simulink model "synchronizing_breaker"  (R2014a)
settings: Solver=FixedStepDiscrete  StartTime=0.0  StopTime=3  FixedStep=Ts  MaxStep=1/60  RelTol=1e-4
PreLoadFcn:
  | load('synchbreaker_data');
StartFcn:
  | tic;
StopFcn:
  | toc;
values from neighbouring files (symbols this model uses):
  d1 = 0.04    [synchbreaker_data.mat]
  Ts = 4e-05    [synchbreaker_data.mat]
libraries: powerlib x11, powerlib_meascontrol x3, simulink x2
settings Model: Creator=gdudgeon  LastModifiedBy=cosorio
settings DataIOCC: SaveOutput=off  SaveTime=off
settings OptimizationCC: ExpressionDepthLimit=2147483647
settings DebuggingCC: UnderspecifiedInitializationDetection=Classic  FcnCallInpInsideContextMsg=UseLocalSettings  StateNameClashWarn=warning
settings SFSimCC: SimParseCustomCode=off
settings GRTTargetCC: CombineOutputUpdateFcns=off  GRTInterface=on

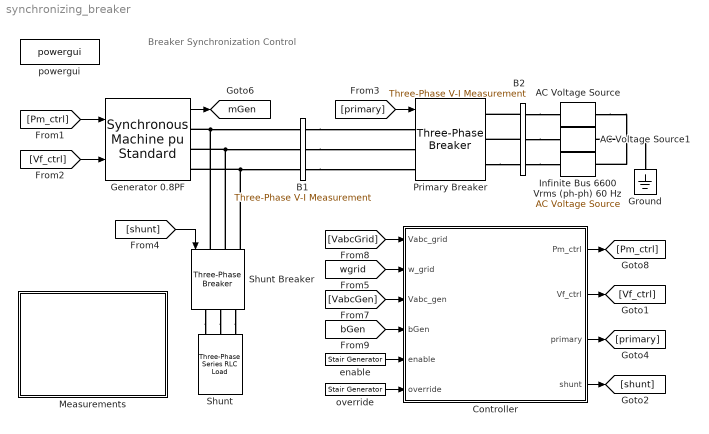
== system synchronizing_breaker ==
  note: Breaker Synchronization Control
  AC Voltage Source : powerlib/Electrical Sources/AC Voltage Source  Amplitude=6600*sqrt(2)/sqrt(3)  Phase=0  Frequency=60  SampleTime=Ts  Measurements=None
  AC Voltage Source1 : powerlib/Electrical Sources/AC Voltage Source  Amplitude=6600*sqrt(2)/sqrt(3)  Phase=-120  Frequency=60  SampleTime=Ts  Measurements=None
  B1 : powerlib/Measurements/Three-Phase V-I Measurement  VoltageMeasurement=phase-to-phase  SetLabelV=on  LabelV=VabcGen  Vpu=off  VpuLL=on  CurrentMeasurement=yes  SetLabelI=on  LabelI=IabcGen  Ipu=on  Pbase=5e6  Vbase=6600  OutputType=Complex  PhasorSimulation=off  PSBequivalent=0
  B2 : powerlib/Measurements/Three-Phase V-I Measurement  VoltageMeasurement=phase-to-phase  SetLabelV=on  LabelV=VabcGrid  Vpu=off  VpuLL=on  CurrentMeasurement=no  SetLabelI=off  LabelI=IabcB2  Ipu=off  Pbase=100e6  Vbase=6600  OutputType=Complex  PhasorSimulation=off  PSBequivalent=0
  Controller : Subsystem  RequirementInfo={'other' 'D:\CVS_Sandbox\P-MLSPG-20171\JIN002 - LPD Modelling\LPD Models\T1702v4_REQM_LINK.doc' '@Simulink_requirement_item_1' 'true' 'Update WR21 automatic synchronisation breaker for use on the LPD model.' '' } %GIDa_fd92f33b_c6ac_4758_9415_28d98727e0ba  TreatAsAtomicUnit=on  SystemSampleTime=Ts
  Generator 0.8PF : powerlib/Machines/Synchronous Machine pu Standard  PresetModel=No  MechanicalLoad=Mechanical power Pm  ShowDetailedParameters=on  RotorType=Salient-pole  Units=per unit standard parameters  MeasurementBus=off  NominalParameters=[5e6 6600 60]  Reactances1=[ 1.81, 0.3, 0.23, 1.76, 0.65, 0.25, 0.15 ]  Reactances2=[1.3050 0.2960 0.2520 0.4740 0.2430 0.1800]  dAxisTimeConstants=Open-circuit  qAxisTimeConstants=Short-circuit  TimeConstants1="[ 4.4849  0.0681  0.1  ]"  TimeConstants2=[ 8.0, 0.03, 1.0, 0.07 ]  TimeConstants3=[4.4900 0.0681 0.0513]  TimeConstants4=[ 8.0, 0.03, 0.3371, 0.0295 ]  TimeConstants5=[ 1.01, 0.053, 0.1 ]  TimeConstants6=[ 1.3201, 0.023, 1.0, 0.07 ]  TimeConstants7=[0.012 0.003 0.003]  TimeConstants8=[ 1.3201, 0.0231, 0.3371, 0.0295 ]  StatorResistance=0.003  Mechanical="[3.7 0.1  4]"  PolePairs=4  InitialConditions=[0 -79.2767 0.4 0.4 0.4 0 -120 120 1.08084]  SetSaturation=off  Saturation=[0.6404,0.7127,0.8441,0.9214,0.9956,1.082,1.19,1.316,1.457;0.7,0.7698,0.8872,0.9466,0.9969,1.046,1.1,1.151,1.201]  LoadFlowParameters=[2 2000000 0 0 0]  TsPowergui=0  TsBlock=-1  IterativeModel=Forward Euler  BusType=swing  Pref=0  Qref=0  Qmin=-inf  Qmax=inf  PLF=0  QLF=0
      settings: AttributesFormatString=%<NominalParameters>
  Ground : powerlib/Elements/Ground  LConnTagsString=a
  Infinite Bus 6600 Vrms (ph-ph) 60 Hz : powerlib/Electrical Sources/AC Voltage Source  Amplitude=6600*sqrt(2)/sqrt(3)  Phase=120  Frequency=60  SampleTime=Ts  Measurements=None
  Measurements : Subsystem
  Primary Breaker : powerlib/Elements/Three-Phase Breaker  InitialState=closed  SwitchA=on  SwitchB=on  SwitchC=on  SwitchTimes="[4/60  10/60]"  External=on  BreakerResistance=1e-5  SnubberResistance=1e6  SnubberCapacitance=Inf  Measurements=None
  Shunt : powerlib/Elements/Three-Phase Series RLC Load  LConnTagsString=A|B|C  Configuration=Y (grounded)  NominalVoltage=6600  NominalFrequency=60  ActivePower=2e5  InductivePower=0  CapacitivePower=0  Measurements=None  LoadType=constant Z
      settings: AttributesFormatString=|
      | P = %<ActivePower> W
      | V = %<NominalVoltage> Vrms
  Shunt Breaker : powerlib/Elements/Three-Phase Breaker  InitialState=open  SwitchA=on  SwitchB=on  SwitchC=on  SwitchTimes="[4/60  10/60]"  External=on  BreakerResistance=1e-5  SnubberResistance=1e6  SnubberCapacitance=Inf  Measurements=None
  enable : powerlib_meascontrol/Pulse & Signal Generators/Stair Generator  t=[0, 1]  e=[0, 1]  Ts=Ts
  override : powerlib_meascontrol/Pulse & Signal Generators/Stair Generator  t=[0, 0.5]  e=[1, 0]  Ts=Ts
  powergui : powerlib/powergui  SimulationMode=Discrete  SolverType=Backward Euler  SampleTime=Ts  frequency=60  SPID=off  DisableSnubberDevices=off  DisableRonSwitches=off  DisableVfSwitches=off  SwTol=0  Interpol=off  DisplayEquations=off  Ts=0  methode=off  frequencyindice=60  Pbase=100e6  ErrMax=1e-4  Iterations=50  UnitsV=kV  UnitsW=MW  FunctionMessages=off  echomessages=off  HookPort=off  EnableUseOfTLC=off  x0status=blocks  RestoreLinks=warning  ResistiveCurrentMeasurement=off  Frange=[0:2:500]  Ylog=off  Xlog=on  ShowGrid=off  save=off  variable=ZData  structure=0  ZoomFFT=on  StartTime=0.0  cycles=1  DisplayStyle=1  fundamental=60  FreqAxis=off  MaxFrequency=1000  frequencyindicesteady=1  RmsSteady=1  display=off
  tag scope: mGen=global
  wires:
  override/1 -> Controller/6(override)
  enable/1 -> Controller/5(enable)
  [Vf_ctrl] -> Generator 0.8PF/2
  [Pm_ctrl] -> Generator 0.8PF/1
  Controller/3(primary) -> [primary]
  [primary] -> Primary Breaker/1
  [shunt] -> Shunt Breaker/1
  Generator 0.8PF/1 -> [mGen]
  [VabcGen] -> Controller/3(Vabc_gen)
  [VabcGrid] -> Controller/1(Vabc_grid)
  [bGen] -> Controller/4(bGen)
  Controller/1(Pm_ctrl) -> [Pm_ctrl]
  Controller/2(Vf_ctrl) -> [Vf_ctrl]
  Controller/4(shunt) -> [shunt]
  [wgrid] -> Controller/2(w_grid)
  connections:
  Shunt Breaker/LConn3 -- B1/LConn3 -- Generator 0.8PF/RConn3
  B2/LConn2 -- Primary Breaker/RConn2
  B1/RConn1 -- Primary Breaker/LConn1
  Shunt Breaker/RConn1 -- Shunt/LConn1
  Shunt Breaker/RConn2 -- Shunt/LConn2
  Shunt Breaker/RConn3 -- Shunt/LConn3
  B2/LConn1 -- Primary Breaker/RConn1
  Shunt Breaker/LConn2 -- B1/LConn2 -- Generator 0.8PF/RConn2
  AC Voltage Source/LConn1 -- Infinite Bus 6600 Vrms (ph-ph) 60 Hz/LConn1 -- Ground/LConn1 -- AC Voltage Source1/LConn1
  B2/RConn1 -- AC Voltage Source/RConn1
  B2/RConn2 -- AC Voltage Source1/RConn1
  B2/RConn3 -- Infinite Bus 6600 Vrms (ph-ph) 60 Hz/RConn1
  Primary Breaker/RConn3 -- B2/LConn3
  B1/RConn2 -- Primary Breaker/LConn2
  Shunt Breaker/LConn1 -- B1/LConn1 -- Generator 0.8PF/RConn1
  B1/RConn3 -- Primary Breaker/LConn3

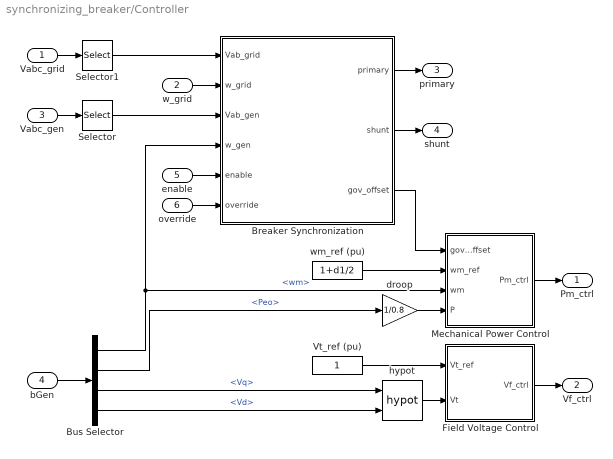
== system synchronizing_breaker/Controller ==
  Vabc_grid : Inport  OutDataTypeStr=double  PortDimensions=3  SampleTime=Ts
  w_grid : Inport  Port=2  OutDataTypeStr=double  PortDimensions=1  SampleTime=Ts
  Vabc_gen : Inport  Port=3  OutDataTypeStr=double  PortDimensions=3  SampleTime=Ts
  bGen : Inport  Port=4  OutDataTypeStr=Bus: GenDataBus
  enable : Inport  Port=5  OutDataTypeStr=double  PortDimensions=1  SampleTime=Ts
  override : Inport  Port=6  OutDataTypeStr=double  PortDimensions=1  SampleTime=Ts
  Breaker Synchronization : Stateflow chart  TreatAsAtomicUnit=on
  Bus Selector : BusSelector  OutputSignals=wm,Peo,Vq,Vd
  Field Voltage Control : Subsystem
  Mechanical Power Control : Subsystem
  Selector : Selector  InputPortWidth=3  Indices=[1]
  Selector1 : Selector  InputPortWidth=3  Indices=[1]
  Vt_ref (pu) : Constant  SampleTime=Ts
  droop : Gain  Gain=1/0.8
  hypot : Math  Operator=hypot  SaturateOnIntegerOverflow=on
  wm_ref (pu) : Constant  Value=1+d1/2  SampleTime=Ts
  Pm_ctrl : Outport  OutDataTypeStr=double  PortDimensions=1  SampleTime=Ts
  Vf_ctrl : Outport  Port=2  OutDataTypeStr=double  PortDimensions=1  SampleTime=Ts
  primary : Outport  Port=3  OutDataTypeStr=double  PortDimensions=1  SampleTime=Ts
  shunt : Outport  Port=4  OutDataTypeStr=double  PortDimensions=1  SampleTime=Ts
  wires:
  override/1 -> Breaker Synchronization/6(override)
  Breaker Synchronization/3(gov_offset) -> Mechanical Power Control/1(gov_offset)
  Breaker Synchronization/1(primary) -> primary/1
  enable/1 -> Breaker Synchronization/5(enable)
  Vabc_gen/1 -> Selector/1
  Selector/1 -> Breaker Synchronization/3(Vab_gen)
  Vabc_grid/1 -> Selector1/1
  Selector1/1 -> Breaker Synchronization/1(Vab_grid)
  Bus Selector/1 -> Mechanical Power Control/3(wm), Breaker Synchronization/4(w_gen)  "<wm>"
  wm_ref (pu)/1 -> Mechanical Power Control/2(wm_ref)
  Mechanical Power Control/1(Pm_ctrl) -> Pm_ctrl/1
  Vt_ref (pu)/1 -> Field Voltage Control/1(Vt_ref)
  Field Voltage Control/1(Vf_ctrl) -> Vf_ctrl/1
  droop/1 -> Mechanical Power Control/4(P)
  bGen/1 -> Bus Selector/1
  hypot/1 -> Field Voltage Control/2(Vt)
  w_grid/1 -> Breaker Synchronization/2(w_grid)
  Bus Selector/2 -> droop/1  "<Peo>"
  Bus Selector/3 -> hypot/1  "<Vq>"
  Bus Selector/4 -> hypot/2  "<Vd>"
  Breaker Synchronization/2(shunt) -> shunt/1

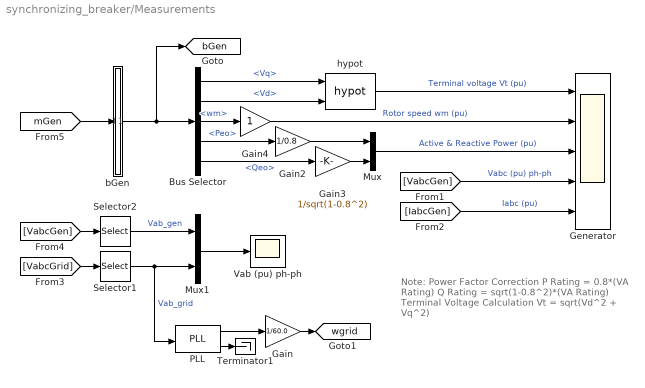
== system synchronizing_breaker/Measurements ==
  note: Note:
      | Power Factor Correction
      | P Rating = 0.8*(VA Rating)
      | Q Rating = sqrt(1-0.8^2)*(VA Rating)
      |
      | Terminal Voltage Calculation
      | Vt = sqrt(Vd^2 + Vq^2)
  Bus Selector : BusSelector  OutputSignals=Vq,Vd,wm,Peo,Qeo
  Gain : Gain  Gain=1/60.0
  Gain2 : Gain  Gain=1/0.8
  Gain3 : Gain  Gain=1/sqrt(1-0.8^2)
  Gain4 : Gain
  Generator : Scope  NumInputPorts=5
      settings: YMin=0.995~0.99~-0.5~-1.5~-0.5  YMax=1.005~1.02~1~1.5~0.5  SaveName=Gen1
  Mux : Mux  Inputs=2
  Mux1 : Mux  Inputs=2
  PLL : powerlib_meascontrol/PLL/PLL  Fmin=45  Par_Init=[0, 60]  ParK=[180, 3200, 1]  TcD=1e-4  MaxRateChangeFreq=12  FilterCutOffFreq=25  Ts=Ts  AGC=on
  Selector1 : Selector  InputPortWidth=3  Indices=[1]
  Selector2 : Selector  InputPortWidth=3  Indices=[1]
  Terminator1 : Terminator
  Vab (pu) ph-ph : Scope
      settings: ShowLegends=on  YMin=-2  YMax=2
  bGen : Subsystem
  hypot : Math  Operator=hypot  SaturateOnIntegerOverflow=on
  tag scope: bGen=global, wgrid=global
  wires:
  hypot/1 -> Generator/1  "Terminal voltage Vt (pu)"
  Mux/1 -> Generator/3  "Active & Reactive Power (pu)"
  [IabcGen] -> Generator/5  "Iabc (pu)"
  [VabcGen] -> Generator/4  "Vabc (pu) ph-ph"
  Gain2/1 -> Mux/1
  Gain3/1 -> Mux/2
  [mGen] -> bGen/1(mGen)
  Bus Selector/1 -> hypot/1  "<Vq>"
  Bus Selector/2 -> hypot/2  "<Vd>"
  Bus Selector/3 -> Gain4/1  "<wm>"
  Bus Selector/4 -> Gain2/1  "<Peo>"
  bGen/1(bGen) -> [bGen], Bus Selector/1
  Bus Selector/5 -> Gain3/1  "<Qeo>"
  Gain4/1 -> Generator/2  "Rotor speed wm (pu)"
  Selector1/1 -> Mux1/2, PLL/1  "Vab_grid"
  PLL/1 -> Gain/1
  PLL/2 -> Terminator1/1
  [VabcGrid] -> Selector1/1
  Gain/1 -> [wgrid]
  [VabcGen] -> Selector2/1
  Selector2/1 -> Mux1/1  "Vab_gen"
  Mux1/1 -> Vab (pu) ph-ph/1

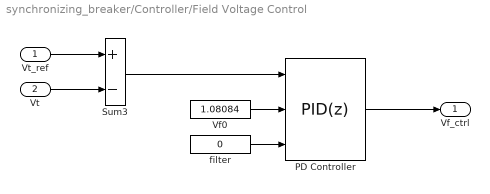
== system synchronizing_breaker/Controller/Field Voltage Control ==
  Vt_ref : Inport
  Vt : Inport  Port=2
  PD Controller : simulink/Continuous/PID Controller  Controller=PID  TimeDomain=Discrete-time  SampleTime=Ts  IntegratorMethod=Forward Euler  FilterMethod=Forward Euler  Form=Parallel  P=200  I=250  D=-1.8  N=100  InitialConditionSource=external  InitialConditionForIntegrator=0  InitialConditionForFilter=0  ExternalReset=none  LimitOutput=off  UpperSaturationLimit=inf  LowerSaturationLimit=-inf  LinearizeAsGain=on  AntiWindupMode=none  Kb=1  TrackingMode=off  Kt=1  PParamMin=[]  PParamMax=[]  IParamMin=[]  IParamMax=[]  DParamMin=[]  DParamMax=[]  NParamMin=[]  NParamMax=[]  KbParamMin=[]  KbParamMax=[]  KtParamMin=[]  KtParamMax=[]  POutMin=[]  POutMax=[]  IOutMin=[]  IOutMax=[]  DOutMin=[]  DOutMax=[]  NOutMin=[]  NOutMax=[]  KbOutMin=[]  KbOutMax=[]  KtOutMin=[]  KtOutMax=[]  IntegratorOutMin=[]  IntegratorOutMax=[]  FilterOutMin=[]  FilterOutMax=[]  SumOutMin=[]  SumOutMax=[]  SumI1OutMin=[]  SumI1OutMax=[]  SumI2OutMin=[]  SumI2OutMax=[]  SumI3OutMin=[]  SumI3OutMax=[]  SumDOutMin=[]  SumDOutMax=[]  SaturationOutMin=[]  SaturationOutMax=[]  IntegratorContinuousStateAttributes=''  IntegratorStateMustResolveToSignalObject=off  IntegratorRTWStateStorageClass=Auto  FilterContinuousStateAttributes=''  FilterStateMustResolveToSignalObject=off  FilterRTWStateStorageClass=Auto
  Sum3 : Sum  Inputs=+-
  Vf0 : Constant  Value=1.08084  SampleTime=Ts
  filter : Constant  Value=0  SampleTime=Ts
  Vf_ctrl : Outport
  wires:
  Sum3/1 -> PD Controller/1
  Vt_ref/1 -> Sum3/1
  Vt/1 -> Sum3/2
  Vf0/1 -> PD Controller/2
  PD Controller/1 -> Vf_ctrl/1
  filter/1 -> PD Controller/3

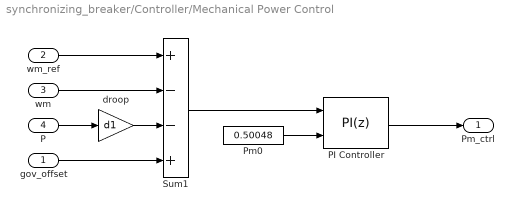
== system synchronizing_breaker/Controller/Mechanical Power Control ==
  gov_offset : Inport
  wm_ref : Inport  Port=2
  wm : Inport  Port=3
  P : Inport  Port=4
  PI Controller : simulink/Continuous/PID Controller  Controller=PI  TimeDomain=Discrete-time  SampleTime=Ts  IntegratorMethod=Forward Euler  FilterMethod=Forward Euler  Form=Parallel  P=400  I=200  D=0.000000000000000  N=99.900066633346043  InitialConditionSource=external  InitialConditionForIntegrator=0  InitialConditionForFilter=0  ExternalReset=none  LimitOutput=off  UpperSaturationLimit=inf  LowerSaturationLimit=-inf  LinearizeAsGain=on  AntiWindupMode=none  Kb=1  TrackingMode=off  Kt=1  PParamMin=[]  PParamMax=[]  IParamMin=[]  IParamMax=[]  DParamMin=[]  DParamMax=[]  NParamMin=[]  NParamMax=[]  KbParamMin=[]  KbParamMax=[]  KtParamMin=[]  KtParamMax=[]  POutMin=[]  POutMax=[]  IOutMin=[]  IOutMax=[]  DOutMin=[]  DOutMax=[]  NOutMin=[]  NOutMax=[]  KbOutMin=[]  KbOutMax=[]  KtOutMin=[]  KtOutMax=[]  IntegratorOutMin=[]  IntegratorOutMax=[]  FilterOutMin=[]  FilterOutMax=[]  SumOutMin=[]  SumOutMax=[]  SumI1OutMin=[]  SumI1OutMax=[]  SumI2OutMin=[]  SumI2OutMax=[]  SumI3OutMin=[]  SumI3OutMax=[]  SumDOutMin=[]  SumDOutMax=[]  SaturationOutMin=[]  SaturationOutMax=[]  IntegratorContinuousStateAttributes=''  IntegratorStateMustResolveToSignalObject=off  IntegratorRTWStateStorageClass=Auto  FilterContinuousStateAttributes=''  FilterStateMustResolveToSignalObject=off  FilterRTWStateStorageClass=Auto
  Pm0 : Constant  Value=0.50048  SampleTime=Ts
  Sum1 : Sum  Inputs=+--+
  droop : Gain  Gain=d1
  Pm_ctrl : Outport
  wires:
  P/1 -> droop/1
  Sum1/1 -> PI Controller/1
  wm_ref/1 -> Sum1/1
  gov_offset/1 -> Sum1/4
  droop/1 -> Sum1/3
  wm/1 -> Sum1/2
  PI Controller/1 -> Pm_ctrl/1
  Pm0/1 -> PI Controller/2

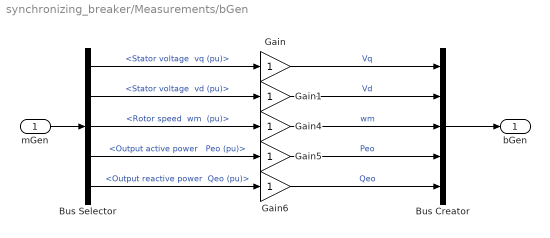
== system synchronizing_breaker/Measurements/bGen ==
  mGen : Inport
  Bus Creator : BusCreator  Inputs=5
  Bus Selector : BusSelector  OutputSignals="dq0 components.Stator voltage  vq (pu),dq0 components.Stator voltage  vd (pu),Mechanical.Rotor speed  wm  (pu),Output active power   Peo (pu),Output reactive power  Qeo (pu)"
  Gain{,1,4..6} (5 alike) : Gain
  bGen : Outport
  wires:
  Gain/1 -> Bus Creator/1  "Vq"
  Bus Selector/1 -> Gain/1  "<Stator voltage  vq (pu)>"
  Bus Selector/2 -> Gain1/1  "<Stator voltage  vd (pu)>"
  Gain1/1 -> Bus Creator/2  "Vd"
  mGen/1 -> Bus Selector/1
  Bus Selector/4 -> Gain5/1  "<Output active power   Peo (pu)>"
  Bus Selector/3 -> Gain4/1  "<Rotor speed  wm  (pu)>"
  Bus Selector/5 -> Gain6/1  "<Output reactive power  Qeo (pu)>"
  Gain4/1 -> Bus Creator/3  "wm"
  Gain6/1 -> Bus Creator/5  "Qeo"
  Gain5/1 -> Bus Creator/4  "Peo"
  Bus Creator/1 -> bGen/1

== stateflow chart synchronizing_breaker/Controller/Breaker Synchronization ==
  settings: updateMethod=DISCRETE  sampleTime=Ts
  state Synchronize
    state PhaseSynch [parallel]
      settings: executionOrder=1
      state InitPhaseSynch
        entry:
        ready = 0;
        primary = 0;
        shunt = 1;
      state Wait
      state PhaseSynchCheck1
        du: Vab_e = Vab_gen - Vab_grid;
      state Connect
        entry:
        ready = 1;
        primary = 1;
        shunt = 0;
      state PhaseSynchCheck2
        du: Vab_e = Vab_gen - Vab_grid;
      (default) -> InitPhaseSynch
      InitPhaseSynch -> Wait : [abs(w_e) < w_tol]
      Wait -> PhaseSynchCheck1 [order 1] : [after(ceil(0.5/Ts),tick)]
      PhaseSynchCheck1 -> Wait [order 1] : [abs(w_e) >= w_tol]
      Wait -> InitPhaseSynch [order 2] : [abs(w_e) >= w_tol]
      PhaseSynchCheck2 -> PhaseSynchCheck1 [order 1] : [abs(Vab_e) >= v_tol]
      PhaseSynchCheck1 -> PhaseSynchCheck2 [order 2] : [abs(Vab_e) < v_tol]
      PhaseSynchCheck2 -> Connect [order 2] : [after(ceil((0.24/60)/Ts),tick) ]
    state FrequencySynch [parallel]
      settings: executionOrder=2
      state InitReadyConnect
        entry:
        gov_offset = 0;
        w_e = 1;
      state SetFrequencyOffset
        during:
        w_e = (w_grid + w_offset) - w_gen;
        y = y_prev+Ts*w_e;
        gov_offset = ki*y + kp*w_e;
        y_prev = y;
      SetFrequencyOffset -> InitReadyConnect : [ready]
      InitReadyConnect -> SetFrequencyOffset : [!ready]
      (default) -> InitReadyConnect
  state Connected
    entry:
    primary = 1;
    shunt = 0;
    gov_offset = 0;
  state Disconnected
    entry:
    primary = 0;
    shunt = 1;
    gov_offset = 0;
  Synchronize -> Connected [order 1] : [override]
  Disconnected -> Synchronize [order 2] : [enable]
  Synchronize -> Disconnected [order 2] : [!enable]
  Connected -> Disconnected : [!override]
  (default) -> Connected
  Disconnected -> Connected [order 1] : [override]
  data: primary output double size=1 =1; shunt output double size=1 =1; Vab_grid input double size=1; w_grid input double size=1; Vab_gen input double size=1; w_gen input double size=1; gov_offset output double =0; Vab_e local double; w_e local double =1; ready local double =0; y local double =0; y_prev local double =0; enable input double size=1; w_offset local double =0.005; ki local double =50; v_tol local double =0.005; w_tol local double =0.005; kp local double =10; override input double size=1; Ts parameter double size=1 =Ts
